simulink model "Matlab2ROS"  (R2023a)
settings: Solver=VariableStepAuto  StartTime=0.0  StopTime=inf  RelTol=1e-3
model workspace (MAT data in the model file):
  Logfile_Data_Object : robotics.ros.BagSelection (value not decoded)
  Logfile_Path = 'D:\Prescan\Documents\Experiments\Custom_scenarios\ROS_Control_for_ModularBus\2024-03-20-17-55-34.bag'
  Logfile_Playback_Duration = nan
  Logfile_Playback_Offset = nan
undefined symbols (not defined in the file or in its folder): Angular, Linear
libraries: robotlib x3, simulink x2
settings Model: Creator=liuhq  LastModifiedBy=liuhq

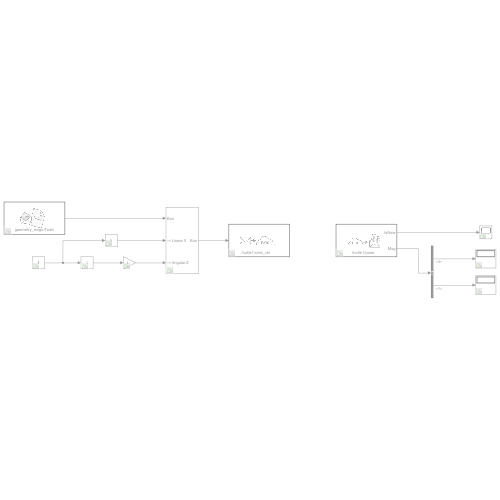
[thumbnail: Simulink's stored preview of the top-level diagram]
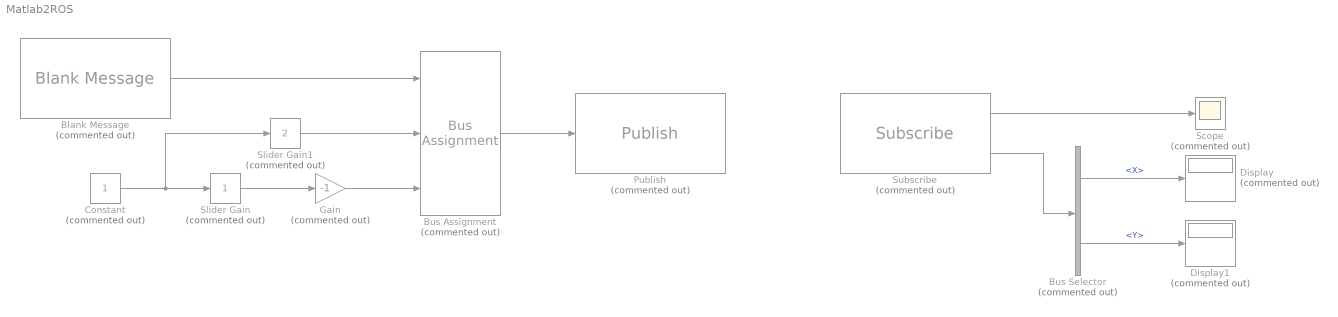
== system Matlab2ROS ==
  Blank Message : robotlib/Blank Message  Commented=on  messageClass=Message  entityType=geometry_msgs/Twist  messageType=geometry_msgs/Twist  SampleTime=-1  legacyBusStruct=off
  Bus Assignment : BusAssignment  Commented=on  AssignedSignals=Linear.X,Angular.Z
  Bus Selector : BusSelector  Commented=on  OutputSignals=X,Y
  Constant : Constant  Commented=on
  Display : Display  Commented=on
  Display1 : Display  Commented=on
  Gain : Gain  Commented=on  Gain=-1
  Publish : robotlib/Publish  Commented=on  topicSource=Select from ROS network  topic=/turtle1/cmd_vel  messageType=geometry_msgs/Twist  legacyBusStruct=off  messageQueueLength=1
  Scope : Scope  Commented=on
  Slider Gain : simulink/Math Operations/Slider Gain  Commented=on  gain=1  low=0  high=2
  Slider Gain1 : simulink/Math Operations/Slider Gain  Commented=on  gain=2  low=0  high=2
  Subscribe : robotlib/Subscribe  Commented=on  topicSource=Select from ROS network  topic=/turtle1/pose  messageType=turtlesim/Pose  SampleTime=-1  legacyBusStruct=off  messageQueueLength=1
  wires:
  Blank Message/1 -> Bus Assignment/1
  Bus Assignment/1 -> Publish/1
  Slider Gain/1 -> Gain/1
  Constant/1 -> Slider Gain1/1, Slider Gain/1
  Slider Gain1/1 -> Bus Assignment/2
  Gain/1 -> Bus Assignment/3
  Subscribe/1 -> Scope/1
  Subscribe/2 -> Bus Selector/1
  Bus Selector/1 -> Display/1  "<X>"
  Bus Selector/2 -> Display1/1  "<Y>"
